simulink model "Inter_connected_tank_simulink"  (R2013a)
settings: Solver=ode45  StartTime=0.0  StopTime=600  RelTol=1e-3
values from neighbouring files (symbols this model uses):
  A = 100    [Inter_connected_tank.m]
  c1 = 4.3    [Inter_connected_tank.m]
  c2 = 6.5    [Inter_connected_tank.m]
  H = 50    [Inter_connected_tank.m]
  R = 18    [Inter_connected_tank.m]
settings Model: Creator=Nima  LastModifiedBy=Nima

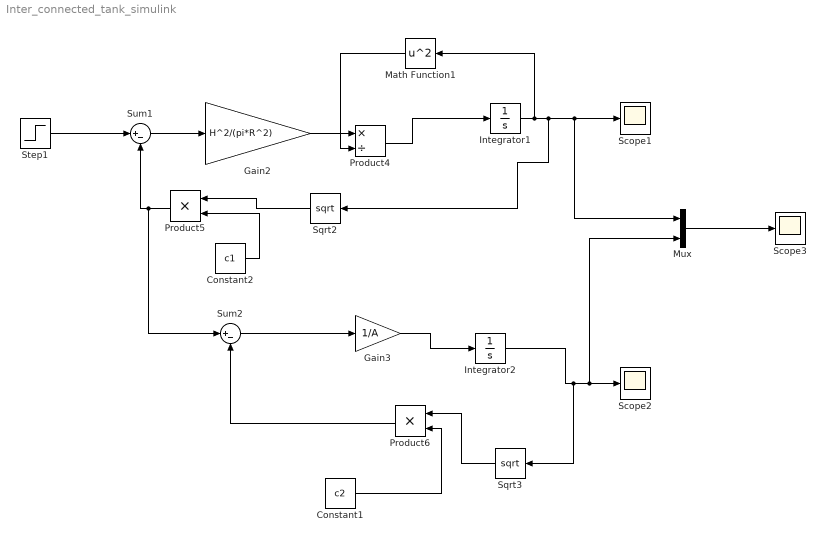
== system Inter_connected_tank_simulink ==
  Constant1 : Constant  Value=c2
  Constant2 : Constant  Value=c1
  Gain2 : Gain  Gain=H^2/(pi*R^2)
  Gain3 : Gain  Gain=1/A
  Integrator1 : Integrator  InitialCondition=0.01  ZeroCross=off
  Integrator2 : Integrator
  Math Function1 : Math  Operator=square  SaturateOnIntegerOverflow=on
  Mux : Mux  Inputs=2
  Product4 : Product  Inputs=*/
  Product5 : Product
  Product6 : Product
  Scope1 : Scope
  Scope2 : Scope
      settings: SaveName=ScopeData2
  Scope3 : Scope
  Sqrt2 : Sqrt  SaturateOnIntegerOverflow=on
  Sqrt3 : Sqrt  SaturateOnIntegerOverflow=on
  Step1 : Step  Before=1  After=13.3  SampleTime=0  ZeroCross=off
  Sum1 : Sum  Inputs=|+-
  Sum2 : Sum  Inputs=|+-
  wires:
  Step1/1 -> Sum1/1
  Sum1/1 -> Gain2/1
  Gain2/1 -> Product4/1
  Math Function1/1 -> Product4/2
  Product4/1 -> Integrator1/1
  Integrator1/1 -> Math Function1/1, Mux/1, Scope1/1, Sqrt2/1
  Sqrt2/1 -> Product5/1
  Product5/1 -> Sum2/1, Sum1/2
  Constant2/1 -> Product5/2
  Sum2/1 -> Gain3/1
  Gain3/1 -> Integrator2/1
  Integrator2/1 -> Sqrt3/1, Mux/2, Scope2/1
  Sqrt3/1 -> Product6/1
  Constant1/1 -> Product6/2
  Product6/1 -> Sum2/2
  Mux/1 -> Scope3/1
